simulink model "deneme5"  (R2023b)
settings: Solver=VariableStepAuto  StartTime=0.0  StopTime=10.0  RelTol=1e-3
model workspace (MAT data in the model file):
  C_torque = 0.0107
values from neighbouring files (symbols this model uses):
  F = [         1, 2, 6, 5 ... (first row only)    [combined_code.m]    (also in spacecraftPoints_v2.m)
undefined symbols (not defined in the file or in its folder): Light, MIL
libraries: aerolibwind2 x1, aerolibpropulsion2 x1, shared6dof x1, aerolibanimutils x1
settings Model: Creator=SafakPC  LastModifiedBy=SafakPC

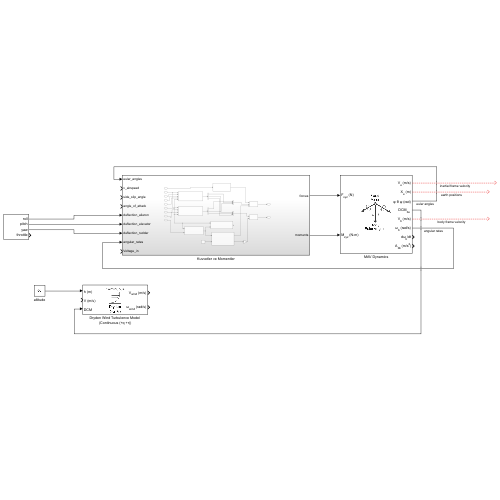
[thumbnail: Simulink's stored preview of the top-level diagram]
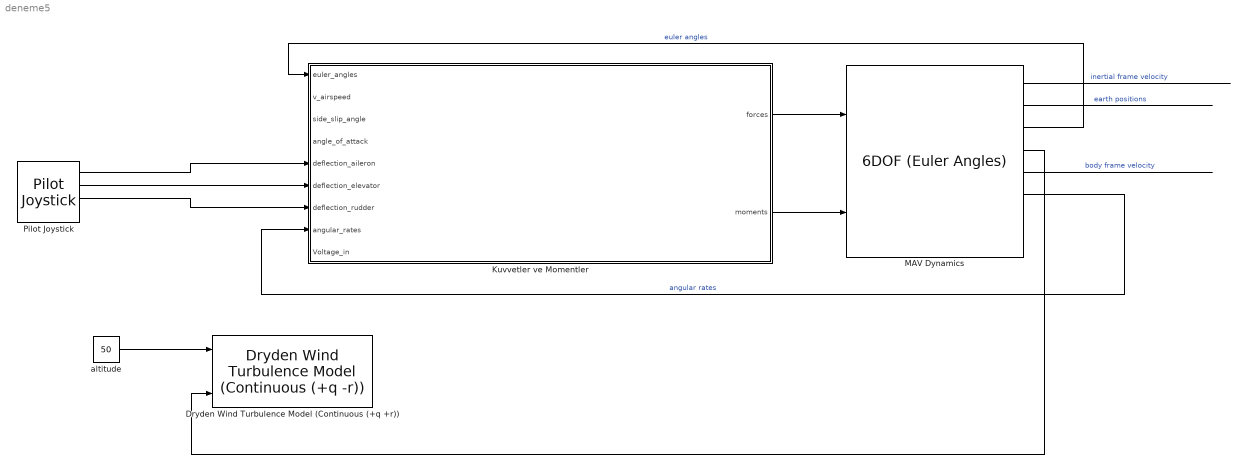
== system deneme5 ==
  Dryden Wind Turbulence Model (Continuous (+q +r)) : aerolibwind2/Dryden Wind Turbulence Model  (Continuous (+q -r))  units=Metric (MKS)  spec=MIL-F-8785C  model=Continuous Dryden (+q +r)  W20=15  Wdeg=0  TurbProb=10^-2 - Light  L_high=533.4  Wingspan=2.9  ts=0.1  Seed=[23341 23342 23343 23344]  T_on=on
      settings: LibrarySourceBlock=|
      | aerolibwind2/Dryden Wind Turbulence Model
      | (Continuous (+q +r))
  Kuvvetler ve Momentler : Subsystem
  MAV Dynamics : shared6dof/6DOF (Euler Angles)  units=Metric (MKS)  mtype=Fixed  rep=Euler Angles  xme_0=[0 0 0]  Vm_0=[0 0 0]  eul_0=[0 0 0]  pm_0=[0 0 0]  mass_0=1.0  mass_e=0.5  mass_f=2.0  inertia=eye(3)  inertia_e=eye(3)  inertia_f=2*eye(3)  k_quat=1.0  vre_flag=on  abi_flag=off  aMode=0  xme_statename=''  Vm_statename=''  eul_statename=''  quat_statename=''  pm_statename=''  mass_statename=''
  Pilot Joystick : aerolibanimutils/Pilot Joystick  JoystickID=Joystick1  OutputConfiguration=FourAxis  SampleTime=1/30
  altitude : Constant  Value=50
  wires:
  Kuvvetler ve Momentler/1(forces) -> MAV Dynamics/1
  Kuvvetler ve Momentler/2(moments) -> MAV Dynamics/2
  MAV Dynamics/3 -> Kuvvetler ve Momentler/1(euler_angles)  "euler angles"
  MAV Dynamics/6 -> Kuvvetler ve Momentler/8(angular_rates)  "angular rates"
  MAV Dynamics/5 -> ?  "body frame velocity"
  MAV Dynamics/1 -> ?  "inertial frame velocity"
  MAV Dynamics/2 -> ?  "earth positions"
  altitude/1 -> Dryden Wind Turbulence Model (Continuous (+q +r))/1
  MAV Dynamics/4 -> Dryden Wind Turbulence Model (Continuous (+q +r))/3
  Pilot Joystick/1 -> Kuvvetler ve Momentler/5(deflection_aileron)
  Pilot Joystick/2 -> Kuvvetler ve Momentler/6(deflection_elevator)
  Pilot Joystick/3 -> Kuvvetler ve Momentler/7(deflection_rudder)

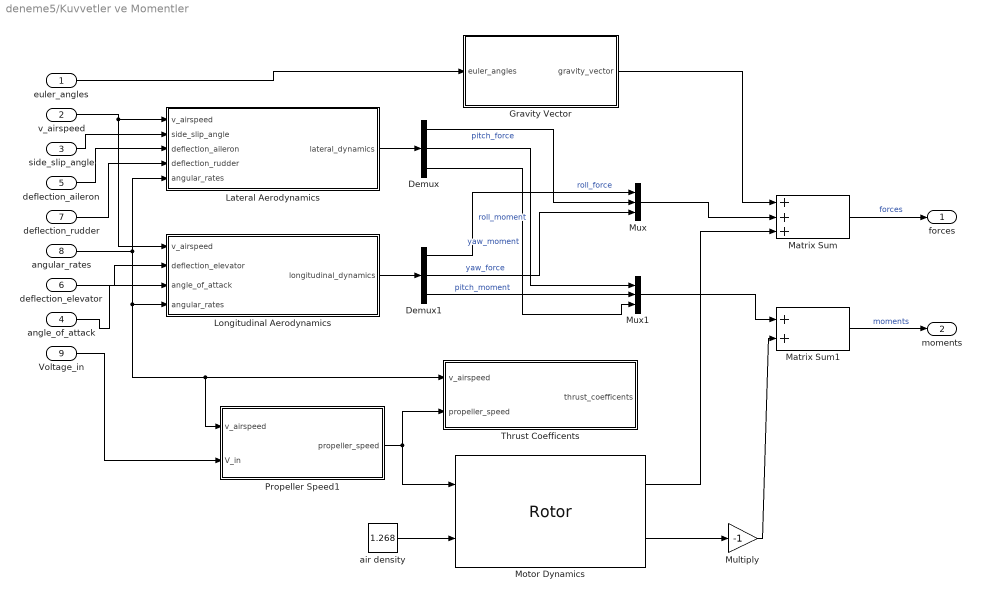
== system deneme5/Kuvvetler ve Momentler ==
  euler_angles : Inport
  v_airspeed : Inport  Port=2
  side_slip_angle : Inport  Port=3
  angle_of_attack : Inport  Port=4
  deflection_aileron : Inport  Port=5
  deflection_elevator : Inport  Port=6
  deflection_rudder : Inport  Port=7
  angular_rates : Inport  Port=8
  Voltage_in : Inport  Port=9
  Demux : Demux  Outputs=3
  Demux1 : Demux  Outputs=3
  Gravity Vector : MATLAB Function  TreatAsAtomicUnit=on
  Lateral Aerodynamics : MATLAB Function  TreatAsAtomicUnit=on
  Longitudinal Aerodynamics : MATLAB Function  TreatAsAtomicUnit=on
  Matrix Sum : Sum  Inputs=+++
  Matrix Sum1 : Sum
  Motor Dynamics : aerolibpropulsion2/Rotor  units=Metric (MKS)  modelMode=Without flap effects  blockSelect=Single  config=Quadcopter X  Nr=1  l=0.0624  h=-0.0159  Arm=[0;0;0]  Nb=2  CTcheck=off  CT=0.0107  CQ=7.8263e-4  CTout=off  R=0.508  c=0.0080  e=0  clalpha=5.5  gamma=0.6051  twistType=Linear  theta0=0.2548  theta1=-0.1361  thetaTip=0.1018  Vb=[0;0;0]  pqr=[0;0;0]
      settings: LibrarySourceBlock=aerolibrotor/Rotor
  Multiply : Gain  Gain=-1
  Mux : Mux  Inputs=3
  Mux1 : Mux  Inputs=3
  Propeller Speed1 : MATLAB Function  TreatAsAtomicUnit=on
  Thrust Coefficents : MATLAB Function  TreatAsAtomicUnit=on
  air density : Constant  Value=1.268
  forces : Outport
  moments : Outport  Port=2
  wires:
  deflection_rudder/1 -> Lateral Aerodynamics/4(deflection_rudder)
  deflection_aileron/1 -> Lateral Aerodynamics/3(deflection_aileron)
  euler_angles/1 -> Gravity Vector/1(euler_angles)
  deflection_elevator/1 -> Longitudinal Aerodynamics/2(deflection_elevator)
  angle_of_attack/1 -> Longitudinal Aerodynamics/3(angle_of_attack)
  Lateral Aerodynamics/1(lateral_dynamics) -> Demux/1
  Demux/1 -> Mux/2  "pitch_force"
  Demux/2 -> Mux1/1  "roll_moment"
  Longitudinal Aerodynamics/1(longitudinal_dynamics) -> Demux1/1
  Demux/3 -> Mux1/3  "yaw_moment"
  Demux1/1 -> Mux/1  "roll_force"
  Demux1/2 -> Mux/3  "yaw_force"
  Demux1/3 -> Mux1/2  "pitch_moment"
  Mux/1 -> Matrix Sum/2
  v_airspeed/1 -> Longitudinal Aerodynamics/1(v_airspeed), Lateral Aerodynamics/1(v_airspeed)
  Gravity Vector/1(gravity_vector) -> Matrix Sum/1
  Matrix Sum/1 -> forces/1  "forces"
  Mux1/1 -> Matrix Sum1/1
  Multiply/1 -> Matrix Sum1/2
  Matrix Sum1/1 -> moments/1  "moments"
  side_slip_angle/1 -> Lateral Aerodynamics/2(side_slip_angle)
  air density/1 -> Motor Dynamics/2
  Propeller Speed1/1(propeller_speed) -> Motor Dynamics/1, Thrust Coefficents/2(propeller_speed)
  angular_rates/1 -> Lateral Aerodynamics/5(angular_rates), Thrust Coefficents/1(v_airspeed), Propeller Speed1/1(v_airspeed), Longitudinal Aerodynamics/4(angular_rates)
  Voltage_in/1 -> Propeller Speed1/2(V_in)
  Motor Dynamics/2 -> Multiply/1
  Motor Dynamics/1 -> Matrix Sum/3

== matlab function deneme5/Kuvvetler ve Momentler/Gravity Vector ==
  data: gravity_vector output; euler_angles input
function gravity_vector = fcn(euler_angles)

    %model parametresi = aerosonde
    mass = 0;

    %yerçekimi vektörünün hesaplanması
    phi = euler_angles(1);
    theta = euler_angles(2);
    psi = euler_angles(3);
    gravity_constant = 9.81;

    a11 = (-mass*gravity_constant*sin(theta));
    a21 = (mass*gravity_constant*cos(theta)*sin(phi));
    a31 = (mass*gravity_constant*cos(theta)*cos(phi));

    gravity_vector = [a11;a21;a31];
    
end

== matlab function deneme5/Kuvvetler ve Momentler/Lateral Aerodynamics ==
  data: v_airspeed input; side_slip_angle input; lateral_dynamics output; deflection_aileron input; deflection_rudder input; angular_rates input
function lateral_dynamics = fcn(v_airspeed, side_slip_angle, deflection_aileron, deflection_rudder, angular_rates)
%model parametreleri - aerosonde
p = angular_rates(1);
r = angular_rates(3);
air_density = 1.268; 
wing_surface_area = 0.55;
wing_span = 2.9; 

CY0 = 0; CYB = -0.83; CYP = 0; CYR = 0; CYDA =  0.075; CYDR = 0.19;
Cl0 = 0; ClB = -0.13; ClP = -0.51; ClR = 0.25; ClDA =0.17; ClDR = 0.0024;
Cn0 = 0; CnB = 0.073; CnP = -0.069; CnR = -0.095; CnDA = -0.011; CnDR = -0.069;

%kuvvet ve momentlerin hesaplanması

var1 = (0.5 * air_density * (v_airspeed^2) * wing_surface_area);
lateral_force = var1 * (CY0 + (CYB*side_slip_angle) + (CYP * ((wing_span/2*v_airspeed)*p))+(CYR * ((wing_span/2*v_airspeed) * r)) + (CYDA * deflection_aileron) + (CYDR * deflection_rudder));
roll_moment = (var1 * wing_span)*(Cl0 + (ClB*side_slip_angle) + (ClP * ((wing_span/2*v_airspeed)*p))+(ClR * ((wing_span/2*v_airspeed) * r)) + (ClDA * deflection_aileron) + (ClDR * deflection_rudder));
yaw_moment = (var1 * wing_span)*(Cn0 + (CnB*side_slip_angle) + (CnP * ((wing_span/2*v_airspeed)*p))+(CnR * ((wing_span/2*v_airspeed) * r)) + (CnDA * deflection_aileron) + (CnDR * deflection_rudder));
lateral_dynamics = [lateral_force;roll_moment;yaw_moment];

end

== matlab function deneme5/Kuvvetler ve Momentler/Longitudinal Aerodynamics ==
  data: v_airspeed input; deflection_elevator input; angle_of_attack input; longitudinal_dynamics output; angular_rates input
function longitudinal_dynamics = fcn(v_airspeed, deflection_elevator, angle_of_attack,   angular_rates)
p = angular_rates(1);
q = angular_rates(2);
r = angular_rates(3);

%model parametereleri - aerosonde
transition_rate = 50; aoa0 = 0.47;
eos = 0.9; CL0 = 0.23; CDp = 0.043; CDq = 0; CLq = 7.95;
CLDe = 0.13; CDDe = 0.0135; 
wing_span =  2.9; wing_surface_area =  0.55;
air_density =  1.268; mean_chord = 0.19;
CM0 = 0.0135; CMa = -2.74; CMq = -38.21 ; CMDe = -0.99;

%lift katsayısının hesaplanması
aspect_ratio = ((wing_span*wing_span) / wing_surface_area);
CL_alpha = (pi*aspect_ratio) / (1+root(1+((aspect_ratio/2)*(aspect_ratio/2))));
CL_flatplate = 2 * sign(angle_of_attack) * sin(angle_of_attack) * sin(angle_of_attack) * cos(angle_of_attack);
var1 = -(transition_rate * (angle_of_attack - aoa0));
var2 = (transition_rate * (angle_of_attack + aoa0));
sigmoid_alpha =  ( 1 + exp(var1) + exp(var2) ) / ( (1 + exp(var1)) * (1 + exp(var2)) );
CL = ((1-sigmoid_alpha)*(CL0 + (angle_of_attack * CL_alpha))) + (sigmoid_alpha*CL_flatplate);

%drag katsayısının hesaplanması
CD = CDp + (((CL_alpha * angle_of_attack)^2) / (pi * eos * aspect_ratio));

%diğer parametrelerin hesaplanması
CX = (-CD * cos(angle_of_attack)) + (CL * sin(angle_of_attack));
CXq = (-CDq * cos(angle_of_attack)) + (CLq * sin(angle_of_attack));
CXDe = (-CDDe * cos(angle_of_attack)) + (CLDe * sin(angle_of_attack));
CZ = (-CD * sin(angle_of_attack)) - (CL * cos(angle_of_attack));
CZq = (-CDq * sin(angle_of_attack)) - (CLq * cos(angle_of_attack));
CZDe = (-CDDe * sin(angle_of_attack)) - (CLDe * cos(angle_of_attack));

%kuvvet ve momentlerin hesaplanması
var1 = (0.5 * air_density * (v_airspeed^2) * wing_surface_area);
roll_force = var1 * (CX + (CXq * ((mean_chord/2*v_airspeed)*q))+ (CXDe * deflection_elevator));
yaw_force = var1 * (CZ + (CZq * ((mean_chord/2*v_airspeed)*q))+ (CZDe * deflection_elevator));
pitch_moment = (var1 *  mean_chord)*(CM0 + (CMa * angle_of_attack) + (CMq * (mean_chord/2*v_airspeed)*q)) + (CMDe * deflection_elevator);
longitudinal_dynamics = [roll_force;yaw_force;pitch_moment];

end

== matlab function deneme5/Kuvvetler ve Momentler/Thrust Coefficents ==
  data: v_airspeed input; thrust_coefficents output; propeller_speed input
function thrust_coefficents = fcn(v_airspeed,propeller_speed)

    %model parametreleri
    prop_diameter = 0.508;
    CT0 =  0.09357; CT1 = -0.06044; CT2 = -0.1079;
    CQ0 =  0.005230; CQ1 =  0.004970; CQ2 = -0.01664;

    J = (2*pi*v_airspeed) / (propeller_speed*prop_diameter);

    C_torque = (CQ2*J*J) + (CQ1*J) + CQ0 ;
    C_thrust = (CT2*J*J) + (CT1*J) + CT0 ; 

    thrust_coefficents = [C_torque;C_thrust];
end

== matlab function deneme5/Kuvvetler ve Momentler/Propeller Speed1 ==
  data: propeller_speed output; v_airspeed input; V_in input
function propeller_speed = fcn(v_airspeed, V_in)

%model parametreleri
air_density = 1.268;
prop_diameter = 0.508;
internal_resistance = 0.042;
no_load_current = 1.5;
KQ = 0.0659; KV = 0.0659; CQ0 = 0.005230; CQ1 = 0.004970; CQ2 = -0.01664;






a = (((air_density * (prop_diameter^5)) / ((2 * pi)*(2 * pi))) * CQ0);
b = ((((air_density * (prop_diameter^4)) / (2*pi)) * (CQ1 * v_airspeed)) + ((KQ*KV) / internal_resistance));
c = (air_density * (prop_diameter^3) * CQ2 * v_airspeed * v_airspeed) - ((KQ/R)*V_in) + (KQ * no_load_current);

omega_P = (-b + sqrt(((b*b)-4*a*c))) / 2*a;

propeller_speed = omega_P;

end
